simulink model "CW_hardware_template"  (R2016b)
settings: Solver=ode5  StartTime=0.0  StopTime=inf  FixedStep=1/100  RelTol=1e-3  AbsTol=1e-6  EnableMultiTasking=on
undefined symbols (not defined in the file): bb, Crane3D_RangeBit, Crane3D_ScaleCoeff, F, G, H, J, L, RTDAC4PCIBaseAddress, Ts, xTarget
(part 11 of 11)

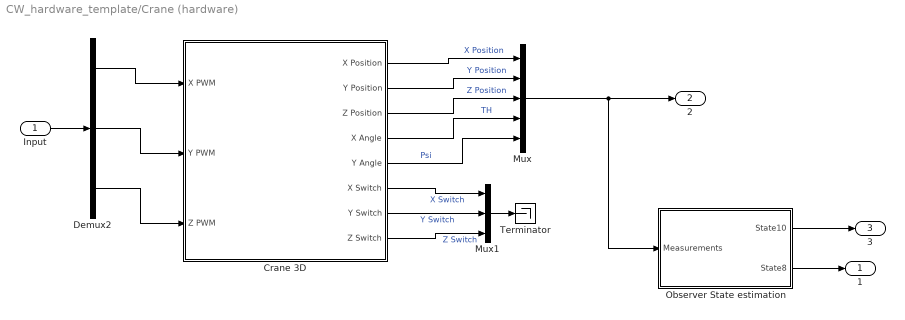
== system CW_hardware_template/Crane (hardware) ==
  Input : Inport
  Crane 3D : Subsystem  mask{BaseAddress=RTDAC4PCIBaseAddress, T0=1/100}
      mask prompts: BaseAddress "Base Address:"; T0 "Sampling Period:"
      mask Display: image(imread('crane.jpeg'))
  Demux2 : Demux  Outputs=3
  Mux : Mux  Inputs=5
  Mux1 : Mux  Inputs=3
  Observer State estimation : Subsystem
  Terminator : Terminator
  1 : Outport
  2 : Outport  Port=2
  3 : Outport  Port=3
  wires:
  Input/1 -> Demux2/1
  Crane 3D/1(X Position) -> Mux/1  "X Position"
  Crane 3D/2(Y Position) -> Mux/2  "Y Position"
  Crane 3D/3(Z Position) -> Mux/3  "Z Position"
  Crane 3D/4(X Angle) -> Mux/4  "TH"
  Crane 3D/5(Y Angle) -> Mux/5  "Psi"
  Mux/1 -> 2/1, Observer State estimation/1(Measurements)
  Crane 3D/6(X Switch) -> Mux1/1  "X Switch"
  Crane 3D/7(Y Switch) -> Mux1/2  "Y Switch"
  Crane 3D/8(Z Switch) -> Mux1/3  "Z Switch"
  Demux2/1 -> Crane 3D/1(X PWM)
  Demux2/2 -> Crane 3D/2(Y PWM)
  Demux2/3 -> Crane 3D/3(Z PWM)
  Observer State estimation/2(State8) -> 1/1
  Mux1/1 -> Terminator/1
  Observer State estimation/1(State10) -> 3/1

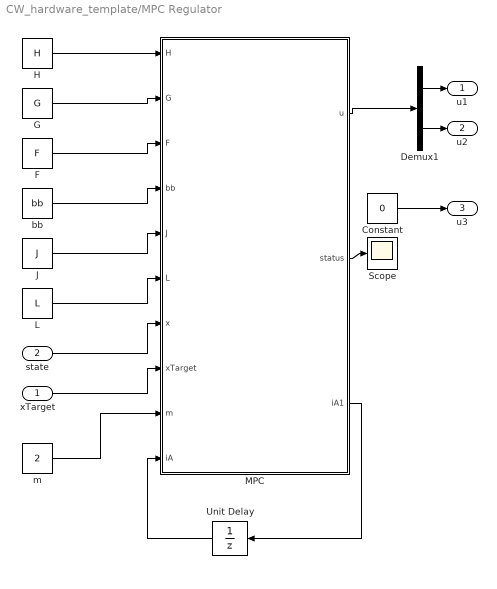
== system CW_hardware_template/MPC Regulator ==
  "xTarget " : Inport
  "state " : Inport  Port=2
  Constant : Constant  Value=0
  Demux1 : Demux  Outputs=2
  F : Constant  Value=F
  G : Constant  Value=G
  H : Constant  Value=H
  J : Constant  Value=J
  L : Constant  Value=L
  MPC : MATLAB Function  TreatAsAtomicUnit=on  SystemSampleTime=Ts
  Scope : Scope
  Unit Delay : UnitDelay  InitialCondition=false(size(bb))  SampleTime=Ts
  bb : Constant  Value=bb
  m : Constant  Value=2
  u1 : Outport
  u2 : Outport  Port=2
  u3 : Outport  Port=3
  wires:
  "state "/1 -> MPC/7(x)
  L/1 -> MPC/6(L)
  MPC/2(status) -> Scope/1
  Demux1/1 -> u1/1
  Demux1/2 -> u2/1
  MPC/1(u) -> Demux1/1
  MPC/3(iA1) -> Unit Delay/1
  Unit Delay/1 -> MPC/10(iA)
  "xTarget "/1 -> MPC/8(xTarget)
  Constant/1 -> u3/1
  H/1 -> MPC/1(H)
  G/1 -> MPC/2(G)
  F/1 -> MPC/3(F)
  bb/1 -> MPC/4(bb)
  J/1 -> MPC/5(J)
  m/1 -> MPC/9(m)

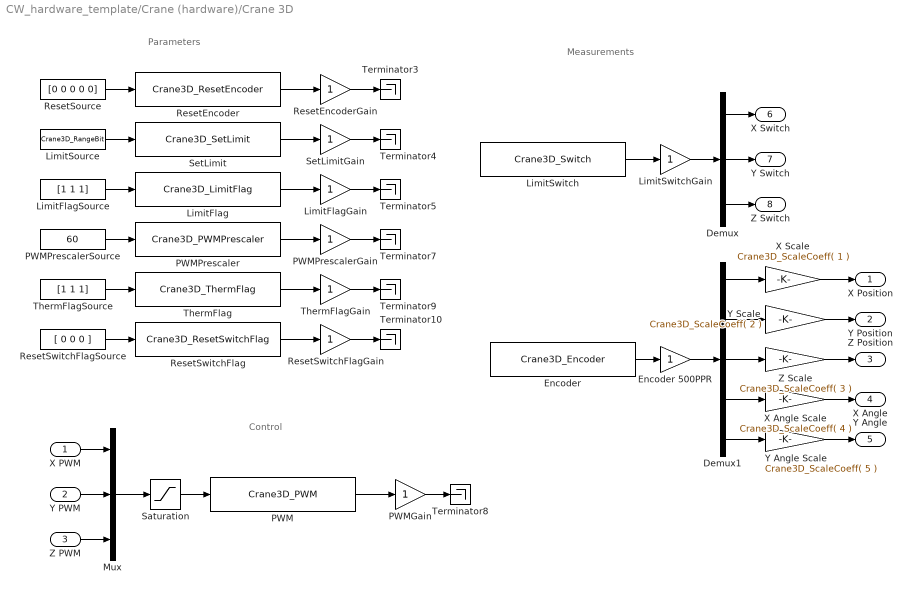
== system CW_hardware_template/Crane (hardware)/Crane 3D ==
  note: Parameters
  note: Control
  note: Measurements
  X PWM : Inport
  Y PWM : Inport  Port=2
  Z PWM : Inport  Port=3
  Demux : Demux  Outputs=3
  Demux1 : Demux  Outputs=5
  Encoder : S-Function  FunctionName=Crane3D_Encoder  Parameters=BaseAddress, T0  SFunctionDeploymentMode=off  EnableBusSupport=off
  Encoder 500PPR : Gain  SaturateOnIntegerOverflow=on  OutDataTypeStr=Inherit: Same as input  ParamDataTypeStr=Inherit: Same as input
  LimitFlag : S-Function  FunctionName=Crane3D_LimitFlag  Parameters=BaseAddress, T0  SFunctionDeploymentMode=off  EnableBusSupport=off
  LimitFlagGain : Gain  SaturateOnIntegerOverflow=on  OutDataTypeStr=Inherit: Same as input  ParamDataTypeStr=Inherit: Same as input
  LimitFlagSource : Constant  Value=[1 1 1]
  LimitSource : Constant  Value=Crane3D_RangeBit
  LimitSwitch : S-Function  FunctionName=Crane3D_Switch  Parameters=BaseAddress, T0  SFunctionDeploymentMode=off  EnableBusSupport=off
  LimitSwitchGain : Gain  SaturateOnIntegerOverflow=on  OutDataTypeStr=Inherit: Same as input  ParamDataTypeStr=Inherit: Same as input
  Mux : Mux  Inputs=3
  PWM : S-Function  FunctionName=Crane3D_PWM  Parameters=BaseAddress, T0  SFunctionDeploymentMode=off  EnableBusSupport=off
  PWMGain : Gain  SaturateOnIntegerOverflow=on  OutDataTypeStr=Inherit: Same as input  ParamDataTypeStr=Inherit: Same as input
  PWMPrescaler : S-Function  FunctionName=Crane3D_PWMPrescaler  Parameters=BaseAddress, T0  SFunctionDeploymentMode=off  EnableBusSupport=off
  PWMPrescalerGain : Gain  SaturateOnIntegerOverflow=on  OutDataTypeStr=Inherit: Same as input  ParamDataTypeStr=Inherit: Same as input
  PWMPrescalerSource : Constant  Value=60
  ResetEncoder : S-Function  FunctionName=Crane3D_ResetEncoder  Parameters=BaseAddress, T0  SFunctionDeploymentMode=off  EnableBusSupport=off
  ResetEncoderGain : Gain  SaturateOnIntegerOverflow=on  OutDataTypeStr=Inherit: Same as input  ParamDataTypeStr=Inherit: Same as input
  ResetSource : Constant  Value=[0 0 0 0 0]
  "ResetSwitchFlag " : S-Function  FunctionName=Crane3D_ResetSwitchFlag  Parameters=BaseAddress, T0  SFunctionDeploymentMode=off  EnableBusSupport=off
  ResetSwitchFlagGain : Gain  SaturateOnIntegerOverflow=on  OutDataTypeStr=Inherit: Same as input  ParamDataTypeStr=Inherit: Same as input
  ResetSwitchFlagSource : Constant  Value=[ 0 0 0 ]
  Saturation : Saturate  UpperLimit=1  LowerLimit=-1
  SetLimit : S-Function  FunctionName=Crane3D_SetLimit  Parameters=BaseAddress, T0  SFunctionDeploymentMode=off  EnableBusSupport=off
  SetLimitGain : Gain  SaturateOnIntegerOverflow=on  OutDataTypeStr=Inherit: Same as input  ParamDataTypeStr=Inherit: Same as input
  Terminator{3..5,7..10} (7 alike) : Terminator
  "ThermFlag " : S-Function  FunctionName=Crane3D_ThermFlag  Parameters=BaseAddress, T0  SFunctionDeploymentMode=off  EnableBusSupport=off
  ThermFlagGain : Gain  SaturateOnIntegerOverflow=on  OutDataTypeStr=Inherit: Same as input  ParamDataTypeStr=Inherit: Same as input
  ThermFlagSource : Constant  Value=[1 1 1]
  X Angle Scale : Gain  Gain=Crane3D_ScaleCoeff( 4 )  OutDataTypeStr=Inherit: Same as input  ParamDataTypeStr=Inherit: Same as input
  X Scale : Gain  Gain=Crane3D_ScaleCoeff( 1 )  OutDataTypeStr=Inherit: Same as input  ParamDataTypeStr=Inherit: Same as input
  Y Angle Scale : Gain  Gain=Crane3D_ScaleCoeff( 5 )  OutDataTypeStr=Inherit: Same as input  ParamDataTypeStr=Inherit: Same as input
  Y Scale : Gain  Gain=Crane3D_ScaleCoeff( 2 )  OutDataTypeStr=Inherit: Same as input  ParamDataTypeStr=Inherit: Same as input
  Z Scale : Gain  Gain=Crane3D_ScaleCoeff( 3 )  OutDataTypeStr=Inherit: Same as input  ParamDataTypeStr=Inherit: Same as input
  X Position : Outport  InitialOutput=0
  Y Position : Outport  Port=2  InitialOutput=0
  Z Position : Outport  Port=3  InitialOutput=0
  X Angle : Outport  Port=4  InitialOutput=0
  Y Angle : Outport  Port=5  InitialOutput=0
  X Switch : Outport  Port=6  InitialOutput=0
  Y Switch : Outport  Port=7  InitialOutput=0
  Z Switch : Outport  Port=8  InitialOutput=0
  wires:
  Encoder 500PPR/1 -> Demux1/1
  Encoder/1 -> Encoder 500PPR/1
  Saturation/1 -> PWM/1
  Mux/1 -> Saturation/1
  PWM/1 -> PWMGain/1
  PWMGain/1 -> Terminator8/1
  ResetEncoder/1 -> ResetEncoderGain/1
  SetLimit/1 -> SetLimitGain/1
  LimitFlag/1 -> LimitFlagGain/1
  PWMPrescaler/1 -> PWMPrescalerGain/1
  "ThermFlag "/1 -> ThermFlagGain/1
  "ResetSwitchFlag "/1 -> ResetSwitchFlagGain/1
  ResetSource/1 -> ResetEncoder/1
  LimitSource/1 -> SetLimit/1
  LimitFlagSource/1 -> LimitFlag/1
  PWMPrescalerSource/1 -> PWMPrescaler/1
  ThermFlagSource/1 -> "ThermFlag "/1
  ResetSwitchFlagSource/1 -> "ResetSwitchFlag "/1
  ResetEncoderGain/1 -> Terminator3/1
  SetLimitGain/1 -> Terminator4/1
  LimitFlagGain/1 -> Terminator5/1
  PWMPrescalerGain/1 -> Terminator7/1
  ThermFlagGain/1 -> Terminator9/1
  ResetSwitchFlagGain/1 -> Terminator10/1
  Z PWM/1 -> Mux/3
  Y PWM/1 -> Mux/2
  X PWM/1 -> Mux/1
  LimitSwitch/1 -> LimitSwitchGain/1
  LimitSwitchGain/1 -> Demux/1
  Demux/1 -> X Switch/1
  Demux/2 -> Y Switch/1
  Demux/3 -> Z Switch/1
  Z Scale/1 -> Z Position/1
  X Scale/1 -> X Position/1
  Y Scale/1 -> Y Position/1
  Y Angle Scale/1 -> Y Angle/1
  X Angle Scale/1 -> X Angle/1
  Demux1/5 -> Y Angle Scale/1
  Demux1/4 -> X Angle Scale/1
  Demux1/3 -> Z Scale/1
  Demux1/2 -> Y Scale/1
  Demux1/1 -> X Scale/1

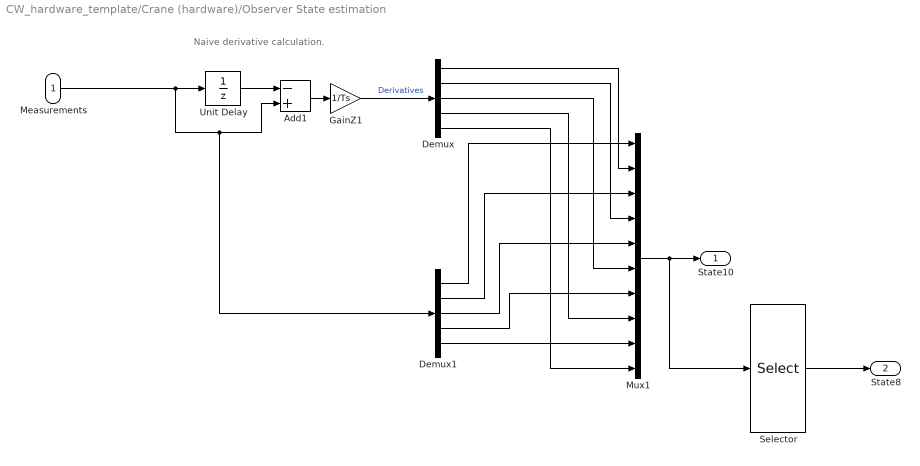
== system CW_hardware_template/Crane (hardware)/Observer State estimation ==
  note: Naive derivative calculation.
  Measurements : Inport
  Add1 : Sum  Inputs=-+
  Demux : Demux  Outputs=5
  Demux1 : Demux  Outputs=5
  GainZ1 : Gain  Gain=1/Ts  SaturateOnIntegerOverflow=on  OutDataTypeStr=Inherit: Same as input  ParamDataTypeStr=Inherit: Same as input
  Mux1 : Mux  Inputs=10
  Selector : Selector  InputPortWidth=10  IndexOptions=Index vector (dialog)  Indices=[1:4 7:10]  OutputSizes=1
  Unit Delay : UnitDelay  InitialCondition="[0.26 0.32 0.3  0 0]"  SampleTime=-1
  State10 : Outport
  State8 : Outport  Port=2
  wires:
  Unit Delay/1 -> Add1/1
  Add1/1 -> GainZ1/1
  Measurements/1 -> Demux1/1, Add1/2, Unit Delay/1
  GainZ1/1 -> Demux/1  "Derivatives"
  Mux1/1 -> Selector/1, State10/1
  Demux1/1 -> Mux1/1
  Demux/1 -> Mux1/2
  Demux1/2 -> Mux1/3
  Demux1/3 -> Mux1/5
  Demux1/4 -> Mux1/7
  Demux1/5 -> Mux1/9
  Demux/2 -> Mux1/4
  Demux/3 -> Mux1/6
  Demux/4 -> Mux1/8
  Demux/5 -> Mux1/10
  Selector/1 -> State8/1

== matlab function CW_hardware_template/MPC Regulator/MPC ==
  data: H input; G input; u output; F input; bb input; J input; L input; x input; xTarget input; m input; status output; iA input boolean; iA1 output boolean
function [u,status,iA1] = myMPController(H,G,F,bb,J,L,x,xTarget,m,iA)
% H       - quadratic term in the cost function.
% G       - matrix in the linear term in the cost function.
% F       - LHS of the inequalities term.
% bb      - RHS of the inequalities term.
% J       - RHS of inequalities term.
% L       - RHS of inequalities term. Use this to shift constraints around target point
% x       - current state
% xTarget - target equilibrium point.
% m       - Number of inputs.
% iA      - active inequalities, see doc mpcqpsolver
%
% u is the first input vector u_0 in the sequence [u_0; u_1; ...; u_{N-1}]; 
% In other words, u is the value of the receding horizon control law
% evaluated with the current state x0 and target xTarget

% Please read the documentation on mpcqpsolver to understand how it is
% suppose to be used. Use iA and iA1 to pass the active inequality vector 

opt = mpcqpsolverOptions;
opt.IntegrityChecks = false;%% for code generation
opt.FeasibilityTol = 1e-3;
opt.DataType = 'double';
%% your code starts here
f = ((x - xTarget)' * G')';
A = -F;
b = -(bb + J * x + L * xTarget);

[U,status,iA1]=mpcqpsolver(H,f,A,b,[],zeros(0,1),iA,opt);

%% your remaining code here

u = U(1:2);


end

% Remember to copy and paste your code above to the Simulink model.
